simulink model "modelo"  (R2021a)
settings: Solver=VariableStepAuto  StartTime=0.0  StopTime=5  RelTol=1e-3
values from neighbouring files (symbols this model uses):
  A = [  0 1 ;  1  -b/I ]    [Program.m]    (also in modelo.m = [   0  1 ; -(masac+masaa)*g*r/I  -b/I ])
  B = [ Tm/I -peso*r/I -b/I]'    [Program.m]    (also in modelo.m = [ 1 Tm/I ]')
  b = 0.08    [Program.m]    (also in modelo.m)
  C = [1 0]    [Program.m]    (also in modelo.m)
  D = 0    [Program.m]    (also in modelo.m)
  g = 9.8    [Program.m]    (also in modelo.m)
  I = 1    [Program.m]    (also in modelo.m = 0.044)
  masaa = 0.581    [modelo.m]
  masac = 0.40    (= 0.4)    [modelo.m]
  r = 0.600    (= 0.6)    [modelo.m]
  Tm = 1    [Program.m]    (also in modelo.m = 4.1)
libraries: pid_lib x1
settings Model: Creator=Usuario  LastModifiedBy=Usuario

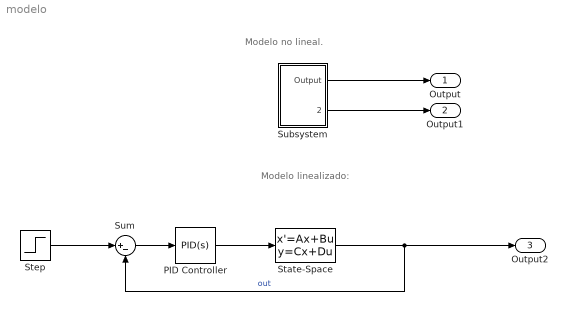
== system modelo ==
  note: Modelo linealizado:
  note: Modelo no lineal.
  PID Controller : pid_lib/PID Controller  Controller=PID  Form=Parallel  TimeDomain=Continuous-time  UseExternalTs=off  SampleTime=-1  IntegratorMethod=Forward Euler  FilterMethod=Forward Euler  ControllerParametersSource=internal  P=6.8700661381378  I=32.9311728475123  D=0.330784848955792  UseFilter=on  N=228.946812421573  TunerSelectOption=Transfer Function Based (PID Tuner App)  InitialConditionSource=internal  InitialConditionForIntegrator=0  InitialConditionForFilter=0  DifferentiatorICPrevScaledInput=0  ExternalReset=none  TrackingMode=off  Kt=1  LimitOutput=off  SatLimitsSource=internal  UpperSaturationLimit=inf  LowerSaturationLimit=-inf  LinearizeAsGain=on  AntiWindupMode=none  Kb=1  POutMin=[]  POutMax=[]  IOutMin=[]  IOutMax=[]  DOutMin=[]  DOutMax=[]  NOutMin=[]  NOutMax=[]  SumOutMin=[]  SumOutMax=[]  SaturationOutMin=[]  SaturationOutMax=[]  PParamMin=[]  PParamMax=[]  IParamMin=[]  IParamMax=[]  DParamMin=[]  DParamMax=[]  NParamMin=[]  NParamMax=[]  KbParamMin=[]  KbParamMax=[]  KtParamMin=[]  KtParamMax=[]  KbOutMin=[]  KbOutMax=[]  KtOutMin=[]  KtOutMax=[]  IntegratorOutMin=[]  IntegratorOutMax=[]  FilterOutMin=[]  FilterOutMax=[]  SumI1OutMin=[]  SumI1OutMax=[]  SumI2OutMin=[]  SumI2OutMax=[]  SumI3OutMin=[]  SumI3OutMax=[]  SumI4OutMin=[]  SumI4OutMax=[]  SumDOutMin=[]  SumDOutMax=[]  DifferentiatorOutMin=[]  DifferentiatorOutMax=[]  FilterDiffOutCoefMin=[]  FilterDiffOutCoefMax=[]  ReciprocalOutMin=[]  ReciprocalOutMax=[]  SumDenOutMin=[]  SumDenOutMax=[]  SumNumOutMin=[]  SumNumOutMax=[]  DivideOutMin=[]  DivideOutMax=[]  UdiffTsProdOutMin=[]  UdiffTsProdOutMax=[]  NTsProdOutMin=[]  NTsProdOutMax=[]  UintegralTsProdOutMin=[]  UintegralTsProdOutMax=[]  UngainTsProdOutMin=[]  UngainTsProdOutMax=[]  IntegratorContinuousStateAttributes=''  IntegratorStateMustResolveToSignalObject=off  IntegratorRTWStateStorageClass=Auto  FilterContinuousStateAttributes=''  FilterStateMustResolveToSignalObject=off  FilterRTWStateStorageClass=Auto  ParallelPVariant=InternalParameters  IdealPVariant=Disabled  IVariant=InternalParameters  DVariant=InternalParameters  IntegratorVariant=Continuous  SatVariant=Disabled  AWVariant=Passthrough  PCopyVariant=Disabled  TRVariant=Disabled  FdbkBlocksVariant=Forward  IdealPFdbkVariant=Disabled  SatFdbkVariant=Disabled  DerivativeFilterVariant=ContFilter  NVariant=InternalParameters  NCopyVariant=Disabled  FilterICVariant=InternalICsFilter  IntegratorICVariant=InternalICs  ExternalResetVariant=Disabled  TRSumVariant=Passthrough  SumFdbkVariant=Disabled  SumVariant=Sum_PID  TsampFilterVariant=InternalTs  TsampNgainVariant=Passthrough  TsampIntegralVariant=Passthrough  ExternalSaturationOutDataTypeStr=Inherit: Same as second input
  State-Space : StateSpace  A=A  B=B  C=C  D=D  InitialCondition=0
  Step : Step  Time=0  SampleTime=0
  Subsystem : Subsystem
  Sum : Sum  Inputs=|+-
  Output : Outport
  Output1 : Outport  Port=2
  Output2 : Outport  Port=3
  wires:
  Subsystem/1(Output) -> Output/1
  Subsystem/2(Output1) -> Output1/1
  State-Space/1 -> Sum/2, Output2/1  "out"
  PID Controller/1 -> State-Space/1
  Step/1 -> Sum/1
  Sum/1 -> PID Controller/1

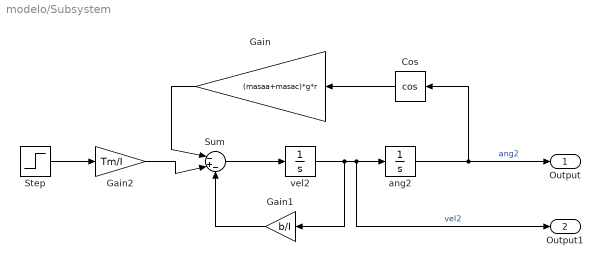
== system modelo/Subsystem ==
  Cos : Trigonometry  Operator=cos
  Gain : Gain  Gain=(masaa+masac)*g*r
  Gain1 : Gain  Gain=b/I
  Gain2 : Gain  Gain=Tm/I
  Step : Step  SampleTime=0
  Sum : Sum  Inputs=|-+-
  ang2 : Integrator  InitialCondition=-0.001
  vel2 : Integrator
  Output : Outport
  Output1 : Outport  Port=2
  wires:
  Gain/1 -> Sum/1
  vel2/1 -> Gain1/1, Output1/1, ang2/1  "vel2"
  Gain1/1 -> Sum/3
  Cos/1 -> Gain/1
  ang2/1 -> Output/1, Cos/1  "ang2"
  Step/1 -> Gain2/1
  Sum/1 -> vel2/1
  Gain2/1 -> Sum/2
